simulink model "MIL_ASW"  (R2019b)
settings: Solver=FixedStepDiscrete  StartTime=0.0  StopTime=2  FixedStep=0.001  RelTol=1e-3  EnableMultiTasking=on
model workspace (MAT data in the model file):
  AccPedlCanVal : Simulink.Signal (value not decoded)
  AccPedlVal : Simulink.Signal (value not decoded)
  BrkPedlCanVal : Simulink.Signal (value not decoded)
  BrkPedlVal : Simulink.Signal (value not decoded)
  Cal1 : Simulink.Parameter (value not decoded)
  Cal10 : Simulink.Parameter (value not decoded)
  Cal11 : Simulink.Parameter (value not decoded)
  Cal12 : Simulink.Parameter (value not decoded)
  Cal2 : Simulink.Parameter (value not decoded)
  Cal3 : Simulink.Parameter (value not decoded)
  Cal4 : Simulink.Parameter (value not decoded)
  Cal5 : Simulink.Parameter (value not decoded)
  Cal6 : Simulink.Parameter (value not decoded)
  Cal7 : Simulink.Parameter (value not decoded)
  Cal8 : Simulink.Parameter (value not decoded)
  Cal9 : Simulink.Parameter (value not decoded)
  Clu1Act : Simulink.Signal (value not decoded)
  Clu1PTar : Simulink.Signal (value not decoded)
  Clu1Req : Simulink.Signal (value not decoded)
  Clu1TqTar : Simulink.Signal (value not decoded)
  Clu2Act : Simulink.Signal (value not decoded)
  Clu2PTar : Simulink.Signal (value not decoded)
  Clu2Req : Simulink.Signal (value not decoded)
  Clu2TqTar : Simulink.Signal (value not decoded)
  CluKissPtPLnch : Simulink.Parameter (value not decoded)
  CluOilTRawVal : Simulink.Signal (value not decoded)
  CluOilTVal : Simulink.Signal (value not decoded)
  CluOpenTqRatMax : Simulink.Parameter (value not decoded)
  CluPMap : Simulink.Parameter (value not decoded)
  CluPMax : Simulink.Parameter (value not decoded)
  CluPMaxGear1 : Simulink.Parameter (value not decoded)
  CluPMaxGear2 : Simulink.Parameter (value not decoded)
  CluPMaxGear3 : Simulink.Parameter (value not decoded)
  CluPMaxGear4 : Simulink.Parameter (value not decoded)
  CluPMaxGear5 : Simulink.Parameter (value not decoded)
  CluPMaxGear6 : Simulink.Parameter (value not decoded)
  CluPMaxGearR : Simulink.Parameter (value not decoded)
  CluPMin : Simulink.Parameter (value not decoded)
  CluPosnMax : Simulink.Parameter (value not decoded)
  CluSoln1IRawVal : Simulink.Signal (value not decoded)
  CluSoln1IReq : Simulink.Signal (value not decoded)
  CluSoln1IReqFlg : Simulink.Signal (value not decoded)
  CluSoln1IVal : Simulink.Signal (value not decoded)
  CluSoln1LineI : Simulink.Parameter (value not decoded)
  CluSoln1LineP : Simulink.Parameter (value not decoded)
  CluSoln1Pwm : Simulink.Signal (value not decoded)
  CluSoln2IRawVal : Simulink.Signal (value not decoded)
  CluSoln2IReq : Simulink.Signal (value not decoded)
  CluSoln2IReqFlg : Simulink.Signal (value not decoded)
  CluSoln2IVal : Simulink.Signal (value not decoded)
  CluSoln2LineI : Simulink.Parameter (value not decoded)
  CluSoln2LineP : Simulink.Parameter (value not decoded)
  CluSoln2Pwm : Simulink.Signal (value not decoded)
  CluTqMap : Simulink.Parameter (value not decoded)
  CrnkSpdRawVal : Simulink.Signal (value not decoded)
  CrnkSpdVal : Simulink.Signal (value not decoded)
  Drive_Intensity_Fuzzy : object (value not decoded)
  DrvIntenFzzy : Simulink.LookupTable (value not decoded)
  EngNIdle : Simulink.Parameter (value not decoded)
  EngNIdleMin : Simulink.Parameter (value not decoded)
  EngSpdCanVal : Simulink.Signal (value not decoded)
  EngThrCanVal : Simulink.Signal (value not decoded)
  EngTqAdd : Simulink.Parameter (value not decoded)
  EngTqCanVal : Simulink.Signal (value not decoded)
  EngTqIntvFlg : Simulink.Signal (value not decoded)
  EngTqIntvRat : Simulink.Signal (value not decoded)
  EngTqMapExtChartc : Simulink.Parameter (value not decoded)
  EngTqMapSpdIndx : Simulink.Parameter (value not decoded)
  EngTqMapThrtIndx : Simulink.Parameter (value not decoded)
  EngTqMapTqMax : Simulink.Parameter (value not decoded)
  EngTqMaxNorm : Simulink.Parameter (value not decoded)
  EngTqRef : Simulink.Parameter (value not decoded)
  EvenCluPRawVal : Simulink.Signal (value not decoded)
  EvenCluPVal : Simulink.Signal (value not decoded)
  EvenInpSpdRawVal : Simulink.Signal (value not decoded)
  EvenInpSpdVal : Simulink.Signal (value not decoded)
  FcnCallTime : Simulink.Parameter (value not decoded)
  FinalRat : Simulink.Parameter (value not decoded)
  Fork1A : Simulink.Parameter (value not decoded)
  Fork1Act : Simulink.Signal (value not decoded)
  Fork1B : Simulink.Parameter (value not decoded)
  Fork1DeltaSpdTar : Simulink.Parameter (value not decoded)
  Fork1MaxSpd1A : Simulink.Parameter (value not decoded)
  Fork1MaxSpd1B : Simulink.Parameter (value not decoded)
  Fork1MaxSpd2A : Simulink.Parameter (value not decoded)
  Fork1MaxSpd2B : Simulink.Parameter (value not decoded)
  Fork1PosnA : Simulink.Parameter (value not decoded)
  Fork1PosnB : Simulink.Parameter (value not decoded)
  Fork1PosnMaxSpd1A : Simulink.Parameter (value not decoded)
  Fork1PosnMaxSpd1B : Simulink.Parameter (value not decoded)
  Fork1PosnMaxSpd2A : Simulink.Parameter (value not decoded)
  Fork1PosnMaxSpd2B : Simulink.Parameter (value not decoded)
  Fork1PosnNeut : Simulink.Parameter (value not decoded)
  Fork1PosnNeutA : Simulink.Parameter (value not decoded)
  Fork1PosnNeutB : Simulink.Parameter (value not decoded)
  Fork1PosnRawVal : Simulink.Signal (value not decoded)
  Fork1PosnSyncA : Simulink.Parameter (value not decoded)
  Fork1PosnSyncB : Simulink.Parameter (value not decoded)
  Fork1PosnVal : Simulink.Signal (value not decoded)
  Fork1SyncTar : Simulink.Parameter (value not decoded)
  Fork2A : Simulink.Parameter (value not decoded)
  Fork2Act : Simulink.Signal (value not decoded)
  Fork2B : Simulink.Parameter (value not decoded)
  Fork2DeltaSpdTar : Simulink.Parameter (value not decoded)
  Fork2MaxSpd1A : Simulink.Parameter (value not decoded)
  Fork2MaxSpd1B : Simulink.Parameter (value not decoded)
  Fork2MaxSpd2A : Simulink.Parameter (value not decoded)
  Fork2MaxSpd2B : Simulink.Parameter (value not decoded)
  Fork2PosnA : Simulink.Parameter (value not decoded)
  Fork2PosnB : Simulink.Parameter (value not decoded)
  Fork2PosnMaxSpd1A : Simulink.Parameter (value not decoded)
  Fork2PosnMaxSpd1B : Simulink.Parameter (value not decoded)
  Fork2PosnMaxSpd2A : Simulink.Parameter (value not decoded)
  Fork2PosnMaxSpd2B : Simulink.Parameter (value not decoded)
  Fork2PosnNeut : Simulink.Parameter (value not decoded)
  Fork2PosnNeutA : Simulink.Parameter (value not decoded)
  Fork2PosnNeutB : Simulink.Parameter (value not decoded)
  Fork2PosnRawVal : Simulink.Signal (value not decoded)
  Fork2PosnSyncA : Simulink.Parameter (value not decoded)
  Fork2PosnSyncB : Simulink.Parameter (value not decoded)
  Fork2PosnVal : Simulink.Signal (value not decoded)
  Fork2SyncTar : Simulink.Parameter (value not decoded)
  Fork3A : Simulink.Parameter (value not decoded)
  Fork3Act : Simulink.Signal (value not decoded)
  Fork3B : Simulink.Parameter (value not decoded)
  Fork3DeltaSpdTar : Simulink.Parameter (value not decoded)
  Fork3MaxSpd1A : Simulink.Parameter (value not decoded)
  Fork3MaxSpd1B : Simulink.Parameter (value not decoded)
  Fork3MaxSpd2A : Simulink.Parameter (value not decoded)
  Fork3MaxSpd2B : Simulink.Parameter (value not decoded)
  Fork3PosnA : Simulink.Parameter (value not decoded)
  Fork3PosnB : Simulink.Parameter (value not decoded)
  Fork3PosnMaxSpd1A : Simulink.Parameter (value not decoded)
  Fork3PosnMaxSpd1B : Simulink.Parameter (value not decoded)
  Fork3PosnMaxSpd2A : Simulink.Parameter (value not decoded)
  Fork3PosnMaxSpd2B : Simulink.Parameter (value not decoded)
  Fork3PosnNeut : Simulink.Parameter (value not decoded)
  Fork3PosnNeutA : Simulink.Parameter (value not decoded)
  Fork3PosnNeutB : Simulink.Parameter (value not decoded)
  Fork3PosnRawVal : Simulink.Signal (value not decoded)
  Fork3PosnSyncA : Simulink.Parameter (value not decoded)
  Fork3PosnSyncB : Simulink.Parameter (value not decoded)
  Fork3PosnVal : Simulink.Signal (value not decoded)
  Fork3SyncTar : Simulink.Parameter (value not decoded)
  Fork4A : Simulink.Parameter (value not decoded)
  Fork4Act : Simulink.Signal (value not decoded)
  Fork4B : Simulink.Parameter (value not decoded)
  Fork4DeltaSpdTar : Simulink.Parameter (value not decoded)
  Fork4MaxSpd1A : Simulink.Parameter (value not decoded)
  Fork4MaxSpd1B : Simulink.Parameter (value not decoded)
  Fork4MaxSpd2A : Simulink.Parameter (value not decoded)
  Fork4MaxSpd2B : Simulink.Parameter (value not decoded)
  Fork4PosnA : Simulink.Parameter (value not decoded)
  Fork4PosnB : Simulink.Parameter (value not decoded)
  Fork4PosnMaxSpd1A : Simulink.Parameter (value not decoded)
  Fork4PosnMaxSpd1B : Simulink.Parameter (value not decoded)
  Fork4PosnMaxSpd2A : Simulink.Parameter (value not decoded)
  Fork4PosnMaxSpd2B : Simulink.Parameter (value not decoded)
  Fork4PosnNeut : Simulink.Parameter (value not decoded)
  Fork4PosnNeutA : Simulink.Parameter (value not decoded)
  Fork4PosnNeutB : Simulink.Parameter (value not decoded)
  Fork4PosnRawVal : Simulink.Signal (value not decoded)
  Fork4PosnSyncA : Simulink.Parameter (value not decoded)
  Fork4PosnSyncB : Simulink.Parameter (value not decoded)
  Fork4PosnVal : Simulink.Signal (value not decoded)
  Fork4SyncTar : Simulink.Parameter (value not decoded)
  FrntWhlRd : Simulink.Parameter (value not decoded)
  GearIdx : Simulink.Parameter (value not decoded)
  GearMax : Simulink.Parameter (value not decoded)
  GearRat : Simulink.Parameter (value not decoded)
  Launch_Engage_Fuzzy : object (value not decoded)
  LnchEngmtFzzy : Simulink.LookupTable (value not decoded)
  LubeSolnIRawVal : Simulink.Signal (value not decoded)
  LubeSolnIReq : Simulink.Signal (value not decoded)
  LubeSolnIVal : Simulink.Signal (value not decoded)
  LubeSolnLineI : Simulink.Parameter (value not decoded)
  LubeSolnLineP : Simulink.Parameter (value not decoded)
  LubeSolnPwm : Simulink.Signal (value not decoded)
  MaiLineSolnIRawVal : Simulink.Signal (value not decoded)
  MaiLineSolnIReq : Simulink.Signal (value not decoded)
  MaiLineSolnIVal : Simulink.Signal (value not decoded)
  MaiLineSolnLineI : Simulink.Parameter (value not decoded)
  MaiLineSolnLineP : Simulink.Parameter (value not decoded)
  MaiLineSolnPwm : Simulink.Signal (value not decoded)
  OddCluPRawVal : Simulink.Signal (value not decoded)
  OddCluPVal : Simulink.Signal (value not decoded)
  OddInpSpdRawVal : Simulink.Signal (value not decoded)
  OddInpSpdVal : Simulink.Signal (value not decoded)
  OutpSpdRawVal : Simulink.Signal (value not decoded)
  OutpSpdVal : Simulink.Signal (value not decoded)
  PsnsrLineP : Simulink.Parameter (value not decoded)
  PsnsrLineV : Simulink.Parameter (value not decoded)
  SftLvrCanVal : Simulink.Signal (value not decoded)
  SftLvrCfm : Simulink.Signal (value not decoded)
  SftLvrVal : Simulink.Signal (value not decoded)
  Shaft1GearAct : Simulink.Signal (value not decoded)
  Shaft1GearReq : Simulink.Signal (value not decoded)
  Shaft2GearAct : Simulink.Signal (value not decoded)
  Shaft2GearReq : Simulink.Signal (value not decoded)
  ShiftMux1SwtReq : Simulink.Signal (value not decoded)
  ShiftMux2SwtReq : Simulink.Signal (value not decoded)
  ShiftSdlEcoDwnSeln : Simulink.Parameter (value not decoded)
  ShiftSdlEcoDwnShift : Simulink.Parameter (value not decoded)
  ShiftSdlEcoUpSeln : Simulink.Parameter (value not decoded)
  ShiftSdlEcoUpShift : Simulink.Parameter (value not decoded)
  ShiftSdlPwrDwnSeln : Simulink.Parameter (value not decoded)
  ShiftSdlPwrDwnShift : Simulink.Parameter (value not decoded)
  ShiftSdlPwrUpSeln : Simulink.Parameter (value not decoded)
  ShiftSdlPwrUpShift : Simulink.Parameter (value not decoded)
  ShiftSdlSACDwnSeln : Simulink.Parameter (value not decoded)
  ShiftSdlSACDwnShift : Simulink.Parameter (value not decoded)
  ShiftSdlSACUpSeln : Simulink.Parameter (value not decoded)
  ShiftSdlSACUpShift : Simulink.Parameter (value not decoded)
  ShiftSdlThrPedlIdx : Simulink.Parameter (value not decoded)
  ShiftSoln1IRawVal : Simulink.Signal (value not decoded)
  ShiftSoln1IReq : Simulink.Signal (value not decoded)
  ShiftSoln1IVal : Simulink.Signal (value not decoded)
  ShiftSoln1LineI : Simulink.Parameter (value not decoded)
  ShiftSoln1LineP : Simulink.Parameter (value not decoded)
  ShiftSoln1Pwm : Simulink.Signal (value not decoded)
  ShiftSoln2IRawVal : Simulink.Signal (value not decoded)
  ShiftSoln2IReq : Simulink.Signal (value not decoded)
  ShiftSoln2IVal : Simulink.Signal (value not decoded)
  ShiftSoln2LineI : Simulink.Parameter (value not decoded)
  ShiftSoln2LineP : Simulink.Parameter (value not decoded)
  ShiftSoln2Pwm : Simulink.Signal (value not decoded)
  SolnOutpTRawVal : Simulink.Signal (value not decoded)
  SolnOutpTVal : Simulink.Signal (value not decoded)
  TSnsr1LineR : Simulink.Parameter (value not decoded)
  TSnsr2LineR : Simulink.Parameter (value not decoded)
  TrsmNrGearAct : Simulink.Signal (value not decoded)
  TrsmNrGearReq : Simulink.Signal (value not decoded)
  TrsmNrPreGearAct : Simulink.Signal (value not decoded)
  TrsmNrPreGearReq : Simulink.Signal (value not decoded)
  Tsnsr1LineT : Simulink.Parameter (value not decoded)
  Tsnsr2LineT : Simulink.Parameter (value not decoded)
  VehSpdCanVal : Simulink.Signal (value not decoded)
  VehSpdTrsmEstimd : Simulink.Signal (value not decoded)
  VehSpdVal : Simulink.Signal (value not decoded)
  VlvBodyTRawVal : Simulink.Signal (value not decoded)
  VlvBodyTVal : Simulink.Signal (value not decoded)
symbols that are objects in the model workspace (value not decoded): CluPMap, CluSoln1LineI, CluSoln1LineP, CluSoln2LineI, CluSoln2LineP, CluTqMap, EngNIdle, EngNIdleMin, EngTqMapThrtIndx, EngTqMapTqMax, EngTqMaxNorm, FcnCallTime, FinalRat, Fork1A, Fork1B, Fork1DeltaSpdTar, Fork1PosnA, Fork1PosnB, Fork1PosnMaxSpd1A, Fork1PosnMaxSpd1B, Fork1PosnMaxSpd2A, Fork1PosnMaxSpd2B, Fork1PosnNeut, Fork1PosnNeutA, Fork1PosnNeutB, Fork1PosnSyncA, Fork1PosnSyncB, Fork1SyncTar, Fork2A, Fork2B, Fork2DeltaSpdTar, Fork2PosnA, Fork2PosnB, Fork2PosnMaxSpd1A, Fork2PosnMaxSpd1B, Fork2PosnMaxSpd2A, Fork2PosnMaxSpd2B, Fork2PosnNeut, Fork2PosnNeutA, Fork2PosnNeutB, Fork2PosnSyncA, Fork2PosnSyncB, Fork2SyncTar, Fork3A, Fork3B, Fork3DeltaSpdTar, Fork3PosnA, Fork3PosnB, Fork3PosnMaxSpd1A, Fork3PosnMaxSpd1B, Fork3PosnMaxSpd2A, Fork3PosnMaxSpd2B, Fork3PosnNeut, Fork3PosnNeutA, Fork3PosnNeutB, Fork3PosnSyncA, Fork3PosnSyncB, Fork3SyncTar, Fork4A, Fork4B
undefined symbols (not defined in the file or in its folder): in1, out1
libraries: simulink x44, fuzblock x3
(part 7 of 10)

== stateflow chart MIL_ASW/Application_Software_SHAW/ASW_ClutchControl_new/Clutch_Control_Strategy ==
  state Inten=Driver_Intention_Fuzzy(AccPeld) [function] [commented out]
  state TqNew=Launch_Applied_Fuzzy(TqOld,Inten,EngN,CluN) [function]
  state Tq = Launch_Torque_Target(EngThr) [function]
  state Tq = Close_Torque_Target(EngThr) [function]
  state Odd_up_to_Even
    state Input [parallel]
      % states initialized
      en:
      Clu1Act=1;
      Clu2Act=0;
      Clu1PReqFlg=1;
      Clu2PReqFlg=1;
      Clu1TqTar=Clu1TqCpEstimd;
      Clu2TqTar=0;
      CluTqTarMin=0;
      CluTqTarMax=40000;
      % torque target initialized
      en:
      CluOffTqTar=Clu1TqTar;
      CluOnTqTar=Clu2TqTar;
      % speed allocation
      en,du:
      CluOffN=InpShaft1N;
      CluOnN=InpShaft2N;
      settings: executionOrder=1
      note: Shift from odd gear to even gear,
          | clutch 1 as off-going clutch,
          | clutch 2 as on-coming clutch
    state Main [parallel]
      settings: executionOrder=2
      state Phase_A
        %Preparation
        state Phase_A_On_Coming [parallel]
          settings: executionOrder=2
          state Phase_A_On_Coming1
            %Wait_for_KissPoint
            en:
            CluOnTqTar=1;
          (default) -> Odd_up_to_Even.Main.Phase_A.Phase_A_On_Coming.Phase_A_On_Coming1
        state Phase_A_Off_Going [parallel]
          settings: executionOrder=1
          state Phase_A_Off_Going1
            %release to slip
            en,du:
            CluTqTarMin=0;
            CluTqDec=1000;
            CluOffTqTar=max(CluOffTqTar-CluTqDec,CluTqTarMin);
          state Phase_A_Off_Going2
            en,du:
            CluTqTarMin=0;
            CluTqDec=100;
            CluOffTqTar=max(CluOffTqTar-CluTqDec,CluTqTarMin);
          state Phase_A_Off_Going3
          (default) -> Odd_up_to_Even.Main.Phase_A.Phase_A_Off_Going.Phase_A_Off_Going1
          Odd_up_to_Even.Main.Phase_A.Phase_A_Off_Going.Phase_A_Off_Going1 -> Odd_up_to_Even.Main.Phase_A.Phase_A_Off_Going.Phase_A_Off_Going2 : [CluOffTqTar<EngTq]
          Odd_up_to_Even.Main.Phase_A.Phase_A_Off_Going.Phase_A_Off_Going2 -> Odd_up_to_Even.Main.Phase_A.Phase_A_Off_Going.Phase_A_Off_Going3 : [abs(EngN-CluOffN)>10]
      state Phase_B_Power_on
        %Torque Phase, Handover
        state Phase_B_On_Coming [parallel]
          settings: executionOrder=1
          state Phase_B_On_Coming1
            en,du:
            CluTqTarMax=EngTq;
            CluTqInc=500;
            CluOnTqTar=min(CluOnTqTar+CluTqInc,CluTqTarMax);
          (default) -> Odd_up_to_Even.Main.Phase_B_Power_on.Phase_B_On_Coming.Phase_B_On_Coming1
        state Phase_B_Off_Going [parallel]
          settings: executionOrder=2
          state Phase_B_Off_Going1
            en,du:
            CluTqTarMin=0;
            CluTqDec=550;
            CluOffTqTar=max(CluOffTqTar-CluTqDec,CluTqTarMin);
          (default) -> Odd_up_to_Even.Main.Phase_B_Power_on.Phase_B_Off_Going.Phase_B_Off_Going1
      state Phase_B_Power_Off
        %Inertia Phase, Handover
        state Phase_B_Off_Going [parallel]
          settings: executionOrder=2
          state Phase_B_Off_Going1
            en,du:
            CluTqTarMin=0;
            CluTqDec=500;
            CluOffTqTar=max(CluOffTqTar-CluTqDec,CluTqTarMin);
          (default) -> Odd_up_to_Even.Main.Phase_B_Power_Off.Phase_B_Off_Going.Phase_B_Off_Going1
        state Phase_B_On_Coming [parallel]
          settings: executionOrder=1
          state Phase_B_On_Coming1
          (default) -> Odd_up_to_Even.Main.Phase_B_Power_Off.Phase_B_On_Coming.Phase_B_On_Coming1
      state Phase_C_Power_on
        %Inertia Phase
        en,du:
        CluTqTarMax=Close_Torque_Target(EngThr);
        CluTqInc=500;
        CluOnTqTar=min(CluOnTqTar+CluTqInc,CluTqTarMax);
      state Phase_C_Power_Off
        %Torque Phase
        en,du:
        CluTqTarMax=Close_Torque_Target(EngThr);
        CluTqInc=500;
        CluOnTqTar=min(CluOnTqTar+CluTqInc,CluTqTarMax);
      state Phase_D_Power_on
        %Synchronization Moment
        en,du:
        CluTqTarMax=Close_Torque_Target(EngThr);
        CluTqInc=500;
        CluOnTqTar=min(CluOnTqTar+CluTqInc,CluTqTarMax);
      state Phase_D_Power_Off
        %Synchronization Moment
        en,du:
        CluTqTarMax=Close_Torque_Target(EngThr);
        CluTqInc=500;
        CluOnTqTar=min(CluOnTqTar+CluTqInc,CluTqTarMax);
      state Phase_E_Power_on
        %Increae pressure for safety
        en,du:
        CluOnTqTar=min(CluOnTqTar+CluTqInc,CluTqTarMax);
        CluTqInc=1000;
        CluTqTarMax=Close_Torque_Target(EngThr);
      state Phase_E_Power_Off
        %Increae pressure for safety
        en,du:
        CluTqTarMax=Close_Torque_Target(EngThr);
        CluTqInc=1000;
        CluOnTqTar=min(CluOnTqTar+CluTqInc,CluTqTarMax);
      state End
      state End1
      (default) -> Odd_up_to_Even.Main.Phase_A
      Odd_up_to_Even.Main.Phase_A -> (junction 335) : [abs(EngN-CluOffN)>10]
      (junction 335) -> (junction 534) [order 2]
      (junction 335) -> Odd_up_to_Even.Main.Phase_B_Power_on [order 1] : [EngN>CluOffN]
          | %Power On
      (junction 534) -> Odd_up_to_Even.Main.Phase_B_Power_Off : %Power off
      Odd_up_to_Even.Main.Phase_B_Power_on -> Odd_up_to_Even.Main.Phase_C_Power_on : [CluOffTqTar<=0&&CluOnTqTar>=CluTqTarMax]
      Odd_up_to_Even.Main.Phase_B_Power_Off -> Odd_up_to_Even.Main.Phase_C_Power_Off : [CluOffTqTar<=0&&EngN<=CluOnN]
      Odd_up_to_Even.Main.Phase_C_Power_on -> Odd_up_to_Even.Main.Phase_D_Power_on : [abs(EngN-CluOnN)<50||...
          | EngN<=CluOnN]
      Odd_up_to_Even.Main.Phase_C_Power_Off -> Odd_up_to_Even.Main.Phase_D_Power_Off : [abs(EngN-CluOnN)<50]
      Odd_up_to_Even.Main.Phase_D_Power_on -> Odd_up_to_Even.Main.Phase_E_Power_on : [abs(EngN-CluOnN)<10]
      Odd_up_to_Even.Main.Phase_D_Power_Off -> Odd_up_to_Even.Main.Phase_E_Power_Off : [abs(EngN-CluOnN)<10]
      Odd_up_to_Even.Main.Phase_E_Power_Off -> Odd_up_to_Even.Main.End1 : [CluOnTqTar>=CluTqTarMax]
      Odd_up_to_Even.Main.Phase_E_Power_on -> Odd_up_to_Even.Main.End : [CluOnTqTar>=CluTqTarMax]
      Odd_up_to_Even.Main.End -> (junction 545)
      Odd_up_to_Even.Main.End1 -> (junction 546)
      (junction 545) -> (junction 546)
    state Output [parallel]
      en,du:
      Clu1TqTar=CluOffTqTar;
      Clu2TqTar=CluOnTqTar;
      settings: executionOrder=3
    (junction 546) -> (junction 859)
  state Odd_down_to_Even
    state Input [parallel]
      % states initialized
      en:
      Clu1Act=1;
      Clu2Act=0;
      Clu1PReqFlg=1;
      Clu2PReqFlg=1;
      Clu1TqTar=Clu1TqCpEstimd;
      Clu2TqTar=0;
      CluTqTarMin=0;
      CluTqTarMax=40000;
      % torque target initialized
      en:
      CluOffTqTar=Clu1TqTar;
      CluOnTqTar=Clu2TqTar;
      % speed allocation
      en,du:
      CluOffN=InpShaft1N;
      CluOnN=InpShaft2N;
      settings: executionOrder=1
      note: Shift from odd gear to even gear,
          | clutch 1 as off-going clutch,
          | clutch 2 as on-coming clutch
    state Main [parallel]
      settings: executionOrder=2
      state Phase_A
        %Preparation
        state Phase_A_Off_Going [parallel]
          settings: executionOrder=1
          state Phase_A_Off_Going1
            %release to slip
            en,du:
            CluTqTarMin=0;
            CluTqDec=1000;
            CluOffTqTar=max(CluOffTqTar-CluTqDec,CluTqTarMin);
          state Phase_A_Off_Going2
            en,du:
            CluTqTarMin=0;
            CluTqDec=100;
            CluOffTqTar=max(CluOffTqTar-CluTqDec,CluTqTarMin);
          state Phase_A_Off_Going3
          (default) -> Odd_down_to_Even.Main.Phase_A.Phase_A_Off_Going.Phase_A_Off_Going1
          Odd_down_to_Even.Main.Phase_A.Phase_A_Off_Going.Phase_A_Off_Going1 -> Odd_down_to_Even.Main.Phase_A.Phase_A_Off_Going.Phase_A_Off_Going2 : [CluOffTqTar<EngTq]
          Odd_down_to_Even.Main.Phase_A.Phase_A_Off_Going.Phase_A_Off_Going2 -> Odd_down_to_Even.Main.Phase_A.Phase_A_Off_Going.Phase_A_Off_Going3 : [abs(EngN-CluOffN)>10]
        state Phase_A_On_Coming [parallel]
          settings: executionOrder=2
          state Phase_A_On_Coming1
            %Wait_for_KissPoint
            en:
            CluOnTqTar=1;
          (default) -> Odd_down_to_Even.Main.Phase_A.Phase_A_On_Coming.Phase_A_On_Coming1
      state Phase_B_Power_on
        %Inertia Phase, Handover
        state Phase_B_Off_Going [parallel]
          settings: executionOrder=2
          state Phase_B_Off_Going1
            en,du:
            CluTqTarMin=0;
            CluTqDec=500;
            CluOffTqTar=max(CluOffTqTar-CluTqDec,CluTqTarMin);
          (default) -> Odd_down_to_Even.Main.Phase_B_Power_on.Phase_B_Off_Going.Phase_B_Off_Going1
        state Phase_B_On_Coming [parallel]
          settings: executionOrder=1
      state Phase_B_Power_Off
        %Torque Phase, Handover
        state Phase_B_Off_Going [parallel]
          settings: executionOrder=2
          state Phase_B_Off_Going1
            en,du:
            CluTqTarMin=0;
            CluTqDec=550;
            CluOffTqTar=max(CluOffTqTar-CluTqDec,CluTqTarMin);
          (default) -> Odd_down_to_Even.Main.Phase_B_Power_Off.Phase_B_Off_Going.Phase_B_Off_Going1
        state Phase_B_On_Coming [parallel]
          settings: executionOrder=1
          state Phase_B_On_Coming1
            en,du:
            CluTqTarMax=Close_Torque_Target(EngThr);
            CluTqInc=500;
            CluOnTqTar=min(CluOnTqTar+CluTqInc,CluTqTarMax);
          (default) -> Odd_down_to_Even.Main.Phase_B_Power_Off.Phase_B_On_Coming.Phase_B_On_Coming1
      state Phase_C_Power_on
        %Torque Phase
        state Phase_C_Off_Going [parallel]
          settings: executionOrder=1
          state Phase_C_Off_Going1
          state Phase_C_Off_Going2
            en,du:
            CluTqTarMin=0;
            CluTqDec=550;
            CluOffTqTar=max(CluOffTqTar-CluTqDec,CluTqTarMin);
          (default) -> Odd_down_to_Even.Main.Phase_C_Power_on.Phase_C_Off_Going.Phase_C_Off_Going1
          Odd_down_to_Even.Main.Phase_C_Power_on.Phase_C_Off_Going.Phase_C_Off_Going1 -> Odd_down_to_Even.Main.Phase_C_Power_on.Phase_C_Off_Going.Phase_C_Off_Going2 : [CluOffTqTar+CluOnTqTar>=EngTq]
        state Phase_C_On_Coming [parallel]
          settings: executionOrder=2
          state Phase_C_On_Coming1
            en,du:
            CluTqTarMax=Close_Torque_Target(EngThr);
            CluTqInc=500;
            CluOnTqTar=min(CluOnTqTar+CluTqInc,CluTqTarMax);
          (default) -> Odd_down_to_Even.Main.Phase_C_Power_on.Phase_C_On_Coming.Phase_C_On_Coming1
      state Phase_C_Power_Off
        %Inertia Phase
        en,du:
        CluTqTarMax=Close_Torque_Target(EngThr);
        CluTqInc=500;
        CluOnTqTar=min(CluOnTqTar+CluTqInc,CluTqTarMax);
      state Phase_D_Power_on
        %Synchronization Moment
        en,du:
        CluTqTarMax=Close_Torque_Target(EngThr);
        CluTqInc=500;
        CluOnTqTar=min(CluOnTqTar+CluTqInc,CluTqTarMax);
      state Phase_D_Power_Off
        %Synchronization Moment
        en,du:
        CluTqTarMax=Close_Torque_Target(EngThr);
        CluTqInc=500;
        CluOnTqTar=min(CluOnTqTar+CluTqInc,CluTqTarMax);
      state Phase_E_Power_on
        %Increae pressure for safety
        en,du:
        CluOnTqTar=min(CluOnTqTar+CluTqInc,CluTqTarMax);
        CluTqInc=1000;
        CluTqTarMax=Close_Torque_Target(EngThr);
      state Phase_E_Power_Off
        %Increae pressure for safety
        en,du:
        CluTqTarMax=Close_Torque_Target(EngThr);
        CluTqInc=1000;
        CluOnTqTar=min(CluOnTqTar+CluTqInc,CluTqTarMax);
      state End
      state End1
      (default) -> Odd_down_to_Even.Main.Phase_A
      Odd_down_to_Even.Main.Phase_A -> (junction 980) : [CluOffTqTar<=0||...
          | abs(EngN-CluOffN)>10]
      (junction 980) -> (junction 981) [order 2]
      (junction 980) -> Odd_down_to_Even.Main.Phase_B_Power_on [order 1] : [EngN>CluOffN]
          | %Power On
      (junction 981) -> Odd_down_to_Even.Main.Phase_B_Power_Off : %Power off
      Odd_down_to_Even.Main.Phase_B_Power_on -> Odd_down_to_Even.Main.Phase_B_Power_Off [order 2] : [EngTq<=0]
          | %change mind
          | % from power-on to power-off
      Odd_down_to_Even.Main.Phase_B_Power_on -> Odd_down_to_Even.Main.Phase_C_Power_on [order 1] : [EngN>CluOnN]
      Odd_down_to_Even.Main.Phase_B_Power_on -> Odd_down_to_Even.Main.Phase_C_Power_on [order 3] : after(100,tick)
      Odd_down_to_Even.Main.Phase_B_Power_Off -> Odd_down_to_Even.Main.Phase_C_Power_Off : [CluOffTqTar<=0]
      Odd_down_to_Even.Main.Phase_C_Power_Off -> Odd_down_to_Even.Main.Phase_D_Power_Off : [abs(EngN-CluOnN)<50]
      Odd_down_to_Even.Main.Phase_C_Power_on -> Odd_down_to_Even.Main.Phase_D_Power_on : [CluOffTqTar<=0&&...
          | abs(EngN-CluOnN)<50]
      Odd_down_to_Even.Main.Phase_D_Power_on -> Odd_down_to_Even.Main.Phase_E_Power_on : [abs(EngN-CluOnN)<10]
      Odd_down_to_Even.Main.Phase_D_Power_Off -> Odd_down_to_Even.Main.Phase_E_Power_Off : [abs(EngN-CluOnN)<10]
      Odd_down_to_Even.Main.Phase_E_Power_Off -> Odd_down_to_Even.Main.End1 : [CluOnTqTar>=CluTqTarMax]
      Odd_down_to_Even.Main.Phase_E_Power_on -> Odd_down_to_Even.Main.End : [CluOnTqTar>=CluTqTarMax]
      Odd_down_to_Even.Main.End -> (junction 982)
      Odd_down_to_Even.Main.End1 -> (junction 954)
      (junction 982) -> (junction 954)
    state Output [parallel]
      en,du:
      Clu1TqTar=CluOffTqTar;
      Clu2TqTar=CluOnTqTar;
      settings: executionOrder=3
    (junction 954) -> (junction 1009)
  state Both_Off_from_Odd2Even
    state Initial
      en:
      Clu1Act=1;
      Clu2Act=0;
      Clu1PReqFlg=1;
      Clu2PReqFlg=1;
      Clu1TqTar=Clu1TqCpEstimd;
      Clu2TqTar=Clu2TqCpEstimd;
    state Phase_A
      state Phase_A_Odd [parallel]
        settings: executionOrder=1
        state Phase_A_Odd
          %release to slip
          en,du:
          CluTqTarMin=0;
          CluTqDec=1000;
          Clu1TqTar=max(Clu1TqTar-CluTqDec,CluTqTarMin);
        state Phase_A_Odd1
          %release clutch
          en,du:
          CluTqTarMin=0;
          CluTqDec=500;
          Clu1TqTar=max(Clu1TqTar-CluTqDec,CluTqTarMin);
        state End
        (default) -> Both_Off_from_Odd2Even.Phase_A.Phase_A_Odd.Phase_A_Odd
        Both_Off_from_Odd2Even.Phase_A.Phase_A_Odd.Phase_A_Odd -> Both_Off_from_Odd2Even.Phase_A.Phase_A_Odd.Phase_A_Odd1 : [abs(EngN-InpShaft1N)>10]
        Both_Off_from_Odd2Even.Phase_A.Phase_A_Odd.Phase_A_Odd1 -> Both_Off_from_Odd2Even.Phase_A.Phase_A_Odd.End : [Clu1TqTar<=0]
      state Phase_A_Even [parallel]
        settings: executionOrder=2
        state Phase_A_Even
          %release to slip
          en,du:
          CluTqTarMin=0;
          CluTqDec=1000;
          Clu2TqTar=max(Clu2TqTar-CluTqDec,CluTqTarMin);
        state Phase_A_Even1
          %release clutch
          en,du:
          CluTqTarMin=0;
          CluTqDec=500;
          Clu2TqTar=max(Clu2TqTar-CluTqDec,CluTqTarMin);
        state End
        (default) -> Both_Off_from_Odd2Even.Phase_A.Phase_A_Even.Phase_A_Even
        Both_Off_from_Odd2Even.Phase_A.Phase_A_Even.Phase_A_Even -> Both_Off_from_Odd2Even.Phase_A.Phase_A_Even.Phase_A_Even1 : [abs(EngN-InpShaft2N)>10]
        Both_Off_from_Odd2Even.Phase_A.Phase_A_Even.Phase_A_Even1 -> Both_Off_from_Odd2Even.Phase_A.Phase_A_Even.End : [Clu2TqTar<=0]
    state End
    (default) -> Both_Off_from_Odd2Even.Initial
    Both_Off_from_Odd2Even.Initial -> Both_Off_from_Odd2Even.Phase_A
    Both_Off_from_Odd2Even.Phase_A -> Both_Off_from_Odd2Even.End : [Clu1TqTar<=0&&Clu2TqTar<=0]
  state Drive_by_Even
    state Initial
      en:
      Clu1Act=0;
      Clu2Act=1;
      Clu1PReqFlg=0;
      Clu2PReqFlg=1;
      Clu1TqTar=0;
      du:
      CluTqTarMax=Close_Torque_Target(EngThr);
      Clu2TqTar=max(Clu2TqTar,CluTqTarMax);
    (default) -> Drive_by_Even.Initial
  state Drive_by_Odd
    state Initial
      en:
      Clu1Act=1;
      Clu2Act=0;
      Clu1PReqFlg=1;
      Clu2PReqFlg=0;
      Clu2TqTar=0;
      du:
      CluTqTarMax=Close_Torque_Target(EngThr);
      Clu1TqTar=max(Clu1TqTar,CluTqTarMax);
    (default) -> Drive_by_Odd.Initial
  state Odd_Off
    state Initial
      en:
      Clu1Act=1;
      Clu2Act=0;
      Clu1PReqFlg=1;
      Clu2PReqFlg=0;
      Clu1TqTar=Clu1TqCpEstimd;
      Clu2TqTar=0;
    state Phase_A
      %release to slip
      en,du:
      CluTqTarMin=0;
      CluTqDec=1000;
      Clu1TqTar=max(Clu1TqTar-CluTqDec,CluTqTarMin);
    state Phase_B
      %release clutch
      en,du:
      CluTqTarMin=0;
      CluTqDec=500;
      Clu1TqTar=max(Clu1TqTar-CluTqDec,CluTqTarMin);
    state End
    (default) -> Odd_Off.Initial
    Odd_Off.Initial -> Odd_Off.Phase_A
    Odd_Off.Phase_A -> Odd_Off.Phase_B : [abs(EngN-InpShaft1N)>10]
    Odd_Off.Phase_B -> Odd_Off.End : [Clu1TqTar<=0]
  state Both_Clutch_Off
    state Keep_Both_off
      en:
      Clu1Act=0;
      Clu2Act=0;
      Clu1PReqFlg=0;
      Clu2PReqFlg=0;
      Clu1TqTar=0;
      Clu2TqTar=0;
      EngTqIntvFlg=0;
      EngTqIntvRat=100;
    (default) -> Keep_Both_off
  state Even_Off
    state Initial
      en:
      Clu1Act=0;
      Clu2Act=1;
      Clu1PReqFlg=0;
      Clu2PReqFlg=1;
      Clu1TqTar=0;
      Clu2TqTar=Clu2TqCpEstimd;
    state Phase_A
      %release to slip
      en,du:
      CluTqTarMin=0;
      CluTqDec=1000;
      Clu2TqTar=max(Clu2TqTar-CluTqDec,CluTqTarMin);
    state Phase_B
      %release clutch
      en,du:
      CluTqTarMin=0;
      CluTqDec=500;
      Clu2TqTar=max(Clu2TqTar-CluTqDec,CluTqTarMin);
    state End
    (default) -> Even_Off.Initial
    Even_Off.Initial -> Even_Off.Phase_A
    Even_Off.Phase_A -> Even_Off.Phase_B : [abs(EngN-InpShaft2N)>10]
    Even_Off.Phase_B -> Even_Off.End : [Clu2TqTar<=0]
  state Odd_On_Process
    state Odd_On
      state Initial
        en:
        Clu1Act=0;
        Clu2Act=0;
        Clu1PReqFlg=1;
        Clu2PReqFlg=0;
        Clu1TqTar=0;
        Clu2TqTar=0;
        CluTqTarMin=0;
        CluTqTarMax=40000;
      state Phase_A
        %Preparation
        %Wait_for_KissPoint
        en:
        Clu1TqTar=1;
      state Phase_B
        %Torque applied
        en,du:
        CluTqTarMax=Close_Torque_Target(EngThr);
        CluTqInc=500;
        Clu1TqTar=min(Clu1TqTar+CluTqInc,CluTqTarMax);
      state Phase_C
        %Synchronization
        en,du:
        CluTqTarMax=Close_Torque_Target(EngThr);
        CluTqInc=500;
        Clu1TqTar=Clu1TqTar+CluTqInc;
      state Phase_D
        %Increae pressure for safety
        en,du:
        CluTqTarMax=Close_Torque_Target(EngThr);
        CluTqInc=1000;
        Clu1TqTar=Clu1TqTar+CluTqInc;
      state End
      (default) -> Odd_On_Process.Odd_On.Initial
      Odd_On_Process.Odd_On.Initial -> Odd_On_Process.Odd_On.Phase_A
      Odd_On_Process.Odd_On.Phase_A -> Odd_On_Process.Odd_On.Phase_B : %[Clu1TqCpEstimd>0]
      Odd_On_Process.Odd_On.Phase_B -> Odd_On_Process.Odd_On.Phase_C : [abs(EngN-InpShaft1N)<50]
      Odd_On_Process.Odd_On.Phase_C -> Odd_On_Process.Odd_On.Phase_D : [abs(EngN-InpShaft1N)<10]
      Odd_On_Process.Odd_On.Phase_D -> Odd_On_Process.Odd_On.End : [Clu1TqTar>=CluTqTarMax]
    state Odd_Launch
      state Initial
        en:
        Clu1Act=0;
        Clu2Act=0;
        Clu1PReqFlg=1;
        Clu2PReqFlg=0;
        Clu1TqTar=0;
        Clu2TqTar=0;
        CluTqTarMin=0;
        CluTqTarMax=40000;
      state Phase_A
        %Preparation
        %Wait_for_KissPoint
        en:
        Clu1TqTar=1;
      state Phase_A1
        %Preparation
        %Wait_for_KissPoint
        en:
        Clu1TqTar=1;
      state Phase_B
        %Torque applied
        en,du:
        CluTqTarMax=Launch_Torque_Target(EngThr);
        %DrvrInten=Driver_Intention_Fuzzy(AccPedl);
        Clu1TqTar=Launch_Applied_Fuzzy(Clu1TqTar,DrvrInten,EngN,InpShaft1N);
        Clu1TqTar=min(Clu1TqTar,CluTqTarMax);
        %CluTqInc=20;
        %Clu1TqTar=min(Clu1TqTar+CluTqInc,CluTqTarMax);
      state Phase_B1
        %Torque applied
        en,du:
        CluTqTarMax=Launch_Torque_Target(EngThr);
        Clu1TqTar=Launch_Applied_Fuzzy(Clu1TqTar,DrvrInten,EngN,InpShaft1N);
        Clu1TqTar=min(Clu1TqTar,CluTqTarMax);
      state Phase_C1
        %Synchronization
        en,du:
        CluTqTarMax=Launch_Torque_Target(EngThr);
        CluTqInc=500;
        Clu1TqTar=Clu1TqTar+CluTqInc;
      state Phase_C
        %Synchronization
        en,du:
        CluTqTarMax=Launch_Torque_Target(EngThr);
        CluTqInc=500;
        Clu1TqTar=Clu1TqTar+CluTqInc;
      state Phase_D
        %Increae pressure for safety
        en,du:
        CluTqTarMax=Launch_Torque_Target(EngThr);
        CluTqInc=1000;
        Clu1TqTar=Clu1TqTar+CluTqInc;
      state Phase_D1
        %Increae pressure for safety
        en,du:
        CluTqTarMax=Launch_Torque_Target(EngThr);
        CluTqInc=1000;
        Clu1TqTar=Clu1TqTar+CluTqInc;
      state End
      state End1
      (default) -> Odd_On_Process.Odd_Launch.Initial
      Odd_On_Process.Odd_Launch.Initial -> Odd_On_Process.Odd_Launch.Phase_A [order 1] : %Static_Launch
          | [VehSpd<200]
      Odd_On_Process.Odd_Launch.Initial -> Odd_On_Process.Odd_Launch.Phase_A1 [order 2] : %Motion_Launch
      Odd_On_Process.Odd_Launch.Phase_A -> Odd_On_Process.Odd_Launch.Phase_B : %[InpShaft1N>0]
      Odd_On_Process.Odd_Launch.Phase_A1 -> Odd_On_Process.Odd_Launch.Phase_B1 : %[InpShaft1N>0]
      Odd_On_Process.Odd_Launch.Phase_B -> Odd_On_Process.Odd_Launch.Phase_C : [EngN>=EngNIdle &&...
          | abs(EngN-InpShaft1N)<50]
      Odd_On_Process.Odd_Launch.Phase_B1 -> Odd_On_Process.Odd_Launch.Phase_C1 : [EngN>=EngNIdle &&...
          | abs(EngN-InpShaft1N)<50]
      Odd_On_Process.Odd_Launch.Phase_C -> Odd_On_Process.Odd_Launch.Phase_D : [abs(EngN-InpShaft1N)<10]
      Odd_On_Process.Odd_Launch.Phase_C1 -> Odd_On_Process.Odd_Launch.Phase_D1 : [abs(EngN-InpShaft1N)<10]
      Odd_On_Process.Odd_Launch.Phase_D -> Odd_On_Process.Odd_Launch.End : [Clu1TqTar>=CluTqTarMax]
      Odd_On_Process.Odd_Launch.Phase_D1 -> Odd_On_Process.Odd_Launch.End1 : [Clu1TqTar>=CluTqTarMax]
      Odd_On_Process.Odd_Launch.End -> (junction 137)
      Odd_On_Process.Odd_Launch.End1 -> (junction 137)
    state Reverse_Launch
      state Initial
        en:
        Clu1Act=0;
        Clu2Act=0;
        Clu1PReqFlg=1;
        Clu2PReqFlg=0;
        Clu1TqTar=0;
        Clu2TqTar=0;
        CluTqTarMin=0;
        CluTqTarMax=40000;
      state Phase_A
        %Preparation
        %Wait_for_KissPoint
        en:
        Clu1TqTar=1;
      state Phase_A1
        %Preparation
        %Wait_for_KissPoint
        en:
        Clu1TqTar=1;
      state Phase_B
        %Torque applied
        en,du:
        CluTqTarMax=Launch_Torque_Target(EngThr);
        Clu1TqTar=Launch_Applied_Fuzzy(Clu1TqTar,DrvrInten,EngN,InpShaft1N);
        Clu1TqTar=min(Clu1TqTar,CluTqTarMax);
      state Phase_B1
        %Torque applied
        en,du:
        CluTqTarMax=Launch_Torque_Target(EngThr);
        Clu1TqTar=Launch_Applied_Fuzzy(Clu1TqTar,DrvrInten,EngN,InpShaft1N);
        Clu1TqTar=min(Clu1TqTar,CluTqTarMax);
      state Phase_C
        %Synchronization
        en,du:
        CluTqTarMax=Close_Torque_Target(EngThr);
        CluTqInc=500;
        Clu1TqTar=Clu1TqTar+CluTqInc;
      state Phase_C1
        %Synchronization
        en,du:
        CluTqTarMax=Close_Torque_Target(EngThr);
        CluTqInc=500;
        Clu1TqTar=Clu1TqTar+CluTqInc;
      state Phase_D
        %Increae pressure for safety
        en,du:
        CluTqTarMax=Launch_Torque_Target(EngThr);
        CluTqInc=1000;
        Clu1TqTar=Clu1TqTar+CluTqInc;
      state Phase_D1
        %Increae pressure for safety
        en,du:
        CluTqTarMax=Launch_Torque_Target(EngThr);
        CluTqInc=1000;
        Clu1TqTar=Clu1TqTar+CluTqInc;
      state End
      state End1
      (default) -> Odd_On_Process.Reverse_Launch.Initial
      Odd_On_Process.Reverse_Launch.Initial -> Odd_On_Process.Reverse_Launch.Phase_A [order 1] : %Static_Launch
          | [VehSpd<200]
      Odd_On_Process.Reverse_Launch.Initial -> Odd_On_Process.Reverse_Launch.Phase_A1 [order 2] : %Motion_Launch
      Odd_On_Process.Reverse_Launch.Phase_A -> Odd_On_Process.Reverse_Launch.Phase_B : %[InpShaft1N>0]
      Odd_On_Process.Reverse_Launch.Phase_A1 -> Odd_On_Process.Reverse_Launch.Phase_B1 : %[InpShaft1N>0]
      Odd_On_Process.Reverse_Launch.Phase_B -> Odd_On_Process.Reverse_Launch.Phase_C : [EngN>=EngNIdle &&...
          | abs(EngN-InpShaft1N)<50]
      Odd_On_Process.Reverse_Launch.Phase_B1 -> Odd_On_Process.Reverse_Launch.Phase_C1 : [EngN>=EngNIdle &&...
          | abs(EngN-InpShaft1N)<50]
      Odd_On_Process.Reverse_Launch.Phase_C1 -> Odd_On_Process.Reverse_Launch.Phase_D1 : [abs(EngN-InpShaft1N)<10]
      Odd_On_Process.Reverse_Launch.Phase_C -> Odd_On_Process.Reverse_Launch.Phase_D : [abs(EngN-InpShaft1N)<10]
      Odd_On_Process.Reverse_Launch.Phase_D -> Odd_On_Process.Reverse_Launch.End : [Clu1TqTar>=CluTqTarMax]
      Odd_On_Process.Reverse_Launch.Phase_D1 -> Odd_On_Process.Reverse_Launch.End1 : [Clu1TqTar>=CluTqTarMax]
      Odd_On_Process.Reverse_Launch.End -> (junction 273)
      Odd_On_Process.Reverse_Launch.End1 -> (junction 273)
  state Even_On_Process
    state Even_On
      state Initial
        en:
        Clu1Act=0;
        Clu2Act=0;
        Clu1PReqFlg=0;
        Clu2PReqFlg=1;
        Clu1TqTar=0;
        Clu2TqTar=0;
        CluTqTarMin=0;
        CluTqTarMax=40000;
      state Phase_A
        %Preparation
        %Wait_for_KissPoint
        en:
        Clu2TqTar=1;
      state Phase_B
        %Torque applied
        en,du:
        CluTqTarMax=Close_Torque_Target(EngThr);
        CluTqInc=500;
        Clu2TqTar=min(Clu2TqTar+CluTqInc,CluTqTarMax);
      state Phase_C
        %Synchronization
        en,du:
        CluTqTarMax=Close_Torque_Target(EngThr);
        CluTqInc=500;
        Clu2TqTar=Clu2TqTar+CluTqInc;
      state Phase_D
        %Increae pressure for safety
        en,du:
        CluTqTarMax=Close_Torque_Target(EngThr);
        CluTqInc=1000;
        Clu2TqTar=Clu2TqTar+CluTqInc;
      state End
      (default) -> Even_On_Process.Even_On.Initial
      Even_On_Process.Even_On.Initial -> Even_On_Process.Even_On.Phase_A
      Even_On_Process.Even_On.Phase_A -> Even_On_Process.Even_On.Phase_B : %[Clu2TqCpEstimd>0]
      Even_On_Process.Even_On.Phase_B -> Even_On_Process.Even_On.Phase_C : [abs(EngN-InpShaft2N)<50]
      Even_On_Process.Even_On.Phase_C -> Even_On_Process.Even_On.Phase_D : [abs(EngN-InpShaft2N)<10]
      Even_On_Process.Even_On.Phase_D -> Even_On_Process.Even_On.End : [Clu2TqTar>=CluTqTarMax]
    state Even_Launch
      state Initial
        en:
        Clu1Act=0;
        Clu2Act=0;
        Clu1PReqFlg=0;
        Clu2PReqFlg=1;
        Clu1TqTar=0;
        Clu2TqTar=0;
        CluTqTarMin=0;
        CluTqTarMax=40000;
      state Phase_A
        %Preparation
        %Wait_for_KissPoint
        en:
        Clu2TqTar=1;
      state Phase_A1
        %Preparation
        %Wait_for_KissPoint
        en:
        Clu2TqTar=1;
      state Phase_B
        %Torque applied
        en,du:
        CluTqTarMax=Launch_Torque_Target(EngThr);
        Clu2TqTar=Launch_Applied_Fuzzy(Clu2TqTar,DrvrInten,EngN,InpShaft2N);
        Clu2TqTar=min(Clu2TqTar,CluTqTarMax);
      state Phase_B1
        %Torque applied
        en,du:
        CluTqTarMax=Launch_Torque_Target(EngThr);
        Clu2TqTar=Launch_Applied_Fuzzy(Clu2TqTar,DrvrInten,EngN,InpShaft2N);
        Clu2TqTar=min(Clu2TqTar+CluTqInc,CluTqTarMax);
      state Phase_C1
        %Synchronization
        en,du:
        CluTqTarMax=Launch_Torque_Target(EngThr);
        CluTqInc=500;
        Clu2TqTar=Clu2TqTar+CluTqInc;
      state Phase_C
        %Synchronization
        en,du:
        CluTqTarMax=Launch_Torque_Target(EngThr);
        CluTqInc=500;
        Clu2TqTar=Clu2TqTar+CluTqInc;
      state Phase_D
        %Increae pressure for safety
        en,du:
        CluTqTarMax=Launch_Torque_Target(EngThr);
        CluTqInc=1000;
        Clu2TqTar=Clu2TqTar+CluTqInc;
      state Phase_D1
        %Increae pressure for safety
        en,du:
        CluTqTarMax=Launch_Torque_Target(EngThr);
        CluTqInc=1000;
        Clu2TqTar=Clu2TqTar+CluTqInc;
      state End
      state End1
      (default) -> Even_On_Process.Even_Launch.Initial
      Even_On_Process.Even_Launch.Initial -> Even_On_Process.Even_Launch.Phase_A [order 1] : %Static_Launch
          | [VehSpd<200]
      Even_On_Process.Even_Launch.Initial -> Even_On_Process.Even_Launch.Phase_A1 [order 2] : %Motion_Launch
      Even_On_Process.Even_Launch.Phase_A -> Even_On_Process.Even_Launch.Phase_B : %[InpShaft2N>0]
      Even_On_Process.Even_Launch.Phase_A1 -> Even_On_Process.Even_Launch.Phase_B1 : %[InpShaft2N>0]
      Even_On_Process.Even_Launch.Phase_B -> Even_On_Process.Even_Launch.Phase_C : [EngN>=EngNIdle &&...
          | abs(EngN-InpShaft2N)<50]
      Even_On_Process.Even_Launch.Phase_B1 -> Even_On_Process.Even_Launch.Phase_C1 : [EngN>=EngNIdle &&...
          | abs(EngN-InpShaft2N)<50]
      Even_On_Process.Even_Launch.Phase_C -> Even_On_Process.Even_Launch.Phase_D : [abs(EngN-InpShaft2N)<10]
      Even_On_Process.Even_Launch.Phase_C1 -> Even_On_Process.Even_Launch.Phase_D1 : [abs(EngN-InpShaft1N)<10]
      Even_On_Process.Even_Launch.Phase_D -> Even_On_Process.Even_Launch.End : [Clu2TqTar>=CluTqTarMax]
      Even_On_Process.Even_Launch.Phase_D1 -> Even_On_Process.Even_Launch.End1 : [Clu2TqTar>=CluTqTarMax]
      Even_On_Process.Even_Launch.End -> (junction 428)
      Even_On_Process.Even_Launch.End1 -> (junction 428)
  state Both_Off_from_Even2Odd
    state Initial
      en:
      Clu1Act=0;
      Clu2Act=1;
      Clu1PReqFlg=1;
      Clu2PReqFlg=1;
      Clu1TqTar=Clu1TqCpEstimd;
      Clu2TqTar=Clu2TqCpEstimd;
    state Phase_A
      state Phase_A_Odd [parallel]
        settings: executionOrder=1
        state Phase_A_Odd
          %release to slip
          en,du:
          CluTqTarMin=0;
          CluTqDec=1000;
          Clu1TqTar=max(Clu1TqTar-CluTqDec,CluTqTarMin);
        state Phase_A_Odd1
          %release clutch
          en,du:
          CluTqTarMin=0;
          CluTqDec=500;
          Clu1TqTar=max(Clu1TqTar-CluTqDec,CluTqTarMin);
        state End
        (default) -> Both_Off_from_Even2Odd.Phase_A.Phase_A_Odd.Phase_A_Odd
        Both_Off_from_Even2Odd.Phase_A.Phase_A_Odd.Phase_A_Odd -> Both_Off_from_Even2Odd.Phase_A.Phase_A_Odd.Phase_A_Odd1 : [abs(EngN-InpShaft1N)>10]
        Both_Off_from_Even2Odd.Phase_A.Phase_A_Odd.Phase_A_Odd1 -> Both_Off_from_Even2Odd.Phase_A.Phase_A_Odd.End : [Clu1TqTar<=0]
      state Phase_A_Even [parallel]
        settings: executionOrder=2
        state Phase_A_Even
          %release to slip
          en,du:
          CluTqTarMin=0;
          CluTqDec=1000;
          Clu2TqTar=max(Clu2TqTar-CluTqDec,CluTqTarMin);
        state Phase_A_Even1
          %release clutch
          en,du:
          CluTqTarMin=0;
          CluTqDec=500;
          Clu2TqTar=max(Clu2TqTar-CluTqDec,CluTqTarMin);
        state End
        (default) -> Both_Off_from_Even2Odd.Phase_A.Phase_A_Even.Phase_A_Even
        Both_Off_from_Even2Odd.Phase_A.Phase_A_Even.Phase_A_Even -> Both_Off_from_Even2Odd.Phase_A.Phase_A_Even.Phase_A_Even1 : [abs(EngN-InpShaft2N)>10]
        Both_Off_from_Even2Odd.Phase_A.Phase_A_Even.Phase_A_Even1 -> Both_Off_from_Even2Odd.Phase_A.Phase_A_Even.End : [Clu2TqTar<=0]
    state End
    (default) -> Both_Off_from_Even2Odd.Initial
    Both_Off_from_Even2Odd.Initial -> Both_Off_from_Even2Odd.Phase_A
    Both_Off_from_Even2Odd.Phase_A -> Both_Off_from_Even2Odd.End : [Clu1TqTar<=0&&Clu2TqTar<=0]
  state Even_up_to_Odd
    state Input [parallel]
      % states initialized
      en:
      Clu1Act=0;
      Clu2Act=1;
      Clu1PReqFlg=1;
      Clu2PReqFlg=1;
      Clu1TqTar=0;
      Clu2TqTar=Clu2TqCpEstimd;
      CluTqTarMin=0;
      CluTqTarMax=40000;
      % torque target initialized
      en:
      CluOffTqTar=Clu2TqTar;
      CluOnTqTar=Clu1TqTar;
      % speed allocation
      en,du:
      CluOffN=InpShaft2N;
      CluOnN=InpShaft1N;
      settings: executionOrder=1
      note: Shift from even gear to odd gear,
          | clutch 1 as on-coming clutch,
          | clutch 2 as off-going clutch
    state Main [parallel]
      settings: executionOrder=2
      state Phase_A
        %Preparation
        state Phase_A_Off_Going [parallel]
          settings: executionOrder=1
          state Phase_A_Off_Going1
            %release to slip
            en,du:
            CluTqTarMin=0;
            CluTqDec=1000;
            CluOffTqTar=max(CluOffTqTar-CluTqDec,CluTqTarMin);
          state Phase_A_Off_Going2
            en,du:
            CluTqTarMin=0;
            CluTqDec=100;
            CluOffTqTar=max(CluOffTqTar-CluTqDec,CluTqTarMin);
          state Phase_A_Off_Going3
          (default) -> Even_up_to_Odd.Main.Phase_A.Phase_A_Off_Going.Phase_A_Off_Going1
          Even_up_to_Odd.Main.Phase_A.Phase_A_Off_Going.Phase_A_Off_Going1 -> Even_up_to_Odd.Main.Phase_A.Phase_A_Off_Going.Phase_A_Off_Going2 : [CluOffTqTar<EngTq]
          Even_up_to_Odd.Main.Phase_A.Phase_A_Off_Going.Phase_A_Off_Going2 -> Even_up_to_Odd.Main.Phase_A.Phase_A_Off_Going.Phase_A_Off_Going3 : [abs(EngN-CluOffN)>10]
        state Phase_A_On_Coming [parallel]
          settings: executionOrder=2
          state Phase_A_On_Coming1
            %Wait_for_KissPoint
            en:
            CluOnTqTar=1;
          (default) -> Even_up_to_Odd.Main.Phase_A.Phase_A_On_Coming.Phase_A_On_Coming1
      state Phase_B_Power_on
        %Torque Phase, Handover
        state Phase_B_On_Coming [parallel]
          settings: executionOrder=1
          state Phase_B_On_Coming1
            en,du:
            CluTqTarMax=EngTq;
            CluTqInc=500;
            CluOnTqTar=min(CluOnTqTar+CluTqInc,CluTqTarMax);
          (default) -> Even_up_to_Odd.Main.Phase_B_Power_on.Phase_B_On_Coming.Phase_B_On_Coming1
        state Phase_B_Off_Going [parallel]
          settings: executionOrder=2
          state Phase_B_Off_Going1
            en,du:
            CluTqTarMin=0;
            CluTqDec=550;
            CluOffTqTar=max(CluOffTqTar-CluTqDec,CluTqTarMin);
          (default) -> Even_up_to_Odd.Main.Phase_B_Power_on.Phase_B_Off_Going.Phase_B_Off_Going1
      state Phase_B_Power_Off
        %Inertia Phase, Handover
        state Phase_B_Off_Going [parallel]
          settings: executionOrder=2
          state Phase_B_Off_Going1
            en,du:
            CluTqTarMin=0;
            CluTqDec=500;
            CluOffTqTar=max(CluOffTqTar-CluTqDec,CluTqTarMin);
          (default) -> Even_up_to_Odd.Main.Phase_B_Power_Off.Phase_B_Off_Going.Phase_B_Off_Going1
        state Phase_B_On_Coming [parallel]
          settings: executionOrder=1
          state Phase_B_On_Coming1
          (default) -> Even_up_to_Odd.Main.Phase_B_Power_Off.Phase_B_On_Coming.Phase_B_On_Coming1
      state Phase_C_Power_on
        %Inertia Phase
        en,du:
        CluTqTarMax=Close_Torque_Target(EngThr);
        CluTqInc=500;
        CluOnTqTar=min(CluOnTqTar+CluTqInc,CluTqTarMax);
      state Phase_C_Power_Off
        %Torque Phase
        en,du:
        CluTqTarMax=Close_Torque_Target(EngThr);
        CluTqInc=500;
        CluOnTqTar=min(CluOnTqTar+CluTqInc,CluTqTarMax);
      state Phase_D_Power_on
        %Synchronization Moment
        en,du:
        CluTqTarMax=Close_Torque_Target(EngThr);
        CluTqInc=500;
        CluOnTqTar=min(CluOnTqTar+CluTqInc,CluTqTarMax);
      state Phase_D_Power_Off
        %Synchronization Moment
        en,du:
        CluTqTarMax=Close_Torque_Target(EngThr);
        CluTqInc=500;
        CluOnTqTar=min(CluOnTqTar+CluTqInc,CluTqTarMax);
      state Phase_E_Power_on
        %Increae pressure for safety
        en,du:
        CluOnTqTar=min(CluOnTqTar+CluTqInc,CluTqTarMax);
        CluTqInc=1000;
        CluTqTarMax=Close_Torque_Target(EngThr);
      state Phase_E_Power_Off
        %Increae pressure for safety
        en,du:
        CluTqTarMax=Close_Torque_Target(EngThr);
        CluTqInc=1000;
        CluOnTqTar=min(CluOnTqTar+CluTqInc,CluTqTarMax);
      state End
      state End1
      (default) -> Even_up_to_Odd.Main.Phase_A
      Even_up_to_Odd.Main.Phase_A -> (junction 912) : [abs(EngN-CluOffN)>10]
      (junction 912) -> (junction 913) [order 2]
      (junction 912) -> Even_up_to_Odd.Main.Phase_B_Power_on [order 1] : [EngN>CluOffN]
          | %Power On
      (junction 913) -> Even_up_to_Odd.Main.Phase_B_Power_Off : %Power off
      Even_up_to_Odd.Main.Phase_B_Power_on -> Even_up_to_Odd.Main.Phase_C_Power_on : [CluOffTqTar<=0&&CluOnTqTar>=CluTqTarMax]
      Even_up_to_Odd.Main.Phase_B_Power_Off -> Even_up_to_Odd.Main.Phase_C_Power_Off : [CluOffTqTar<=0&&EngN<=CluOnN]
      Even_up_to_Odd.Main.Phase_C_Power_on -> Even_up_to_Odd.Main.Phase_D_Power_on : [abs(EngN-CluOnN)<50||...
          | EngN<=CluOnN]
      Even_up_to_Odd.Main.Phase_C_Power_Off -> Even_up_to_Odd.Main.Phase_D_Power_Off : [abs(EngN-CluOnN)<50||...
          | EngN>=CluOnN]
      Even_up_to_Odd.Main.Phase_D_Power_on -> Even_up_to_Odd.Main.Phase_E_Power_on : [abs(EngN-CluOnN)<10]
      Even_up_to_Odd.Main.Phase_D_Power_Off -> Even_up_to_Odd.Main.Phase_E_Power_Off : [abs(EngN-CluOnN)<10]
      Even_up_to_Odd.Main.Phase_E_Power_Off -> Even_up_to_Odd.Main.End1 : [CluOnTqTar>=CluTqTarMax]
      Even_up_to_Odd.Main.Phase_E_Power_on -> Even_up_to_Odd.Main.End : [CluOnTqTar>=CluTqTarMax]
      Even_up_to_Odd.Main.End -> (junction 914)
      Even_up_to_Odd.Main.End1 -> (junction 886)
      (junction 886) -> (junction 914)
    state Output [parallel]
      en,du:
      Clu1TqTar=CluOnTqTar;
      Clu2TqTar=CluOffTqTar;
      settings: executionOrder=3
    (junction 914) -> (junction 585)
  state Even_down_to_Odd
    state Input [parallel]
      % states initialized
      en:
      Clu1Act=0;
      Clu2Act=1;
      Clu1PReqFlg=1;
      Clu2PReqFlg=1;
      Clu1TqTar=0;
      Clu2TqTar=Clu2TqCpEstimd;
      CluTqTarMin=0;
      CluTqTarMax=40000;
      % torque target initialized
      en:
      CluOffTqTar=Clu2TqTar;
      CluOnTqTar=Clu1TqTar;
      % speed allocation
      en,du:
      CluOffN=InpShaft2N;
      CluOnN=InpShaft1N;
      settings: executionOrder=1
      note: Shift from even gear to odd gear,
          | clutch 1 as off-coming clutch,
          | clutch 2 as on-going clutch
    state Main [parallel]
      settings: executionOrder=2
      state Phase_A
        %Preparation
        state Phase_A_Off_Going [parallel]
          settings: executionOrder=1
          state Phase_A_Off_Going1
            %release to slip
            en,du:
            CluTqTarMin=0;
            CluTqDec=1000;
            CluOffTqTar=max(CluOffTqTar-CluTqDec,CluTqTarMin);
          state Phase_A_Off_Going2
            en,du:
            CluTqTarMin=0;
            CluTqDec=100;
            CluOffTqTar=max(CluOffTqTar-CluTqDec,CluTqTarMin);
          state Phase_A_Off_Going3
          (default) -> Even_down_to_Odd.Main.Phase_A.Phase_A_Off_Going.Phase_A_Off_Going1
          Even_down_to_Odd.Main.Phase_A.Phase_A_Off_Going.Phase_A_Off_Going1 -> Even_down_to_Odd.Main.Phase_A.Phase_A_Off_Going.Phase_A_Off_Going2 : [CluOffTqTar<EngTq]
          Even_down_to_Odd.Main.Phase_A.Phase_A_Off_Going.Phase_A_Off_Going2 -> Even_down_to_Odd.Main.Phase_A.Phase_A_Off_Going.Phase_A_Off_Going3 : [abs(EngN-CluOffN)>10]
        state Phase_A_On_Coming [parallel]
          settings: executionOrder=2
          state Phase_A_On_Coming1
            %Wait_for_KissPoint
            en:
            CluOnTqTar=1;
          (default) -> Even_down_to_Odd.Main.Phase_A.Phase_A_On_Coming.Phase_A_On_Coming1
      state Phase_B_Power_on
        %Inertia Phase, Handover
        state Phase_B_Off_Going [parallel]
          settings: executionOrder=2
          state Phase_B_Off_Going1
            en,du:
            CluTqTarMin=0;
            CluTqDec=500;
            CluOffTqTar=max(CluOffTqTar-CluTqDec,CluTqTarMin);
          (default) -> Even_down_to_Odd.Main.Phase_B_Power_on.Phase_B_Off_Going.Phase_B_Off_Going1
        state Phase_B_On_Coming [parallel]
          settings: executionOrder=1
      state Phase_B_Power_Off
        %Torque Phase, Handover
        state Phase_B_Off_Going [parallel]
          settings: executionOrder=2
          state Phase_B_Off_Going1
            en,du:
            CluTqTarMin=0;
            CluTqDec=550;
            CluOffTqTar=max(CluOffTqTar-CluTqDec,CluTqTarMin);
          (default) -> Even_down_to_Odd.Main.Phase_B_Power_Off.Phase_B_Off_Going.Phase_B_Off_Going1
        state Phase_B_On_Coming [parallel]
          settings: executionOrder=1
          state Phase_B_On_Coming1
            en,du:
            CluTqTarMax=Close_Torque_Target(EngThr);
            CluTqInc=500;
            CluOnTqTar=min(Clu2TqTar+CluTqInc,CluTqTarMax);
          (default) -> Even_down_to_Odd.Main.Phase_B_Power_Off.Phase_B_On_Coming.Phase_B_On_Coming1
      state Phase_C_Power_on
        %Torque Phase
        state Phase_C_Off_Going [parallel]
          settings: executionOrder=1
          state Phase_C_Off_Going1
          state Phase_C_Off_Going2
            en,du:
            CluTqTarMin=0;
            CluTqDec=550;
            CluOffTqTar=max(CluOffTqTar-CluTqDec,CluTqTarMin);
          (default) -> Even_down_to_Odd.Main.Phase_C_Power_on.Phase_C_Off_Going.Phase_C_Off_Going1
          Even_down_to_Odd.Main.Phase_C_Power_on.Phase_C_Off_Going.Phase_C_Off_Going1 -> Even_down_to_Odd.Main.Phase_C_Power_on.Phase_C_Off_Going.Phase_C_Off_Going2 : [CluOffTqTar+CluOnTqTar>=EngTq]
        state Phase_C_On_Coming [parallel]
          settings: executionOrder=2
          state Phase_C_On_Coming1
            en,du:
            CluTqTarMax=Close_Torque_Target(EngThr);
            CluTqInc=500;
            CluOnTqTar=min(CluOnTqTar+CluTqInc,CluTqTarMax);
          (default) -> Even_down_to_Odd.Main.Phase_C_Power_on.Phase_C_On_Coming.Phase_C_On_Coming1
      state Phase_C_Power_Off
        %Inertia Phase
        en,du:
        CluTqTarMax=Close_Torque_Target(EngThr);
        CluTqInc=500;
        CluOnTqTar=min(CluOnTqTar+CluTqInc,CluTqTarMax);
      state Phase_D_Power_on
        %Synchronization Moment
        en,du:
        CluTqTarMax=Close_Torque_Target(EngThr);
        CluTqInc=500;
        CluOnTqTar=min(CluOnTqTar+CluTqInc,CluTqTarMax);
      state Phase_D_Power_Off
        %Synchronization Moment
        en,du:
        CluTqTarMax=Close_Torque_Target(EngThr);
        CluTqInc=500;
        CluOnTqTar=min(CluOnTqTar+CluTqInc,CluTqTarMax);
      state Phase_E_Power_on
        %Increae pressure for safety
        en,du:
        CluTqTarMax=Close_Torque_Target(EngThr);
        CluTqInc=1000;
        CluOnTqTar=min(CluOnTqTar+CluTqInc,CluTqTarMax);
      state Phase_E_Power_Off
        %Increae pressure for safety
        en,du:
        CluTqTarMax=Close_Torque_Target(EngThr);
        CluTqInc=1000;
        CluOnTqTar=min(CluOnTqTar+CluTqInc,CluTqTarMax);
      state End
      state End1
      (default) -> Even_down_to_Odd.Main.Phase_A
      Even_down_to_Odd.Main.Phase_A -> (junction 1152) : [CluOffTqTar<=0||...
          | abs(EngN-CluOffN)>10]
      (junction 1152) -> (junction 1147) [order 2]
      (junction 1152) -> Even_down_to_Odd.Main.Phase_B_Power_on [order 1] : [EngN>CluOffN]
          | %Power On
      (junction 1147) -> Even_down_to_Odd.Main.Phase_B_Power_Off : %Power off
      Even_down_to_Odd.Main.Phase_B_Power_on -> Even_down_to_Odd.Main.Phase_B_Power_Off [order 2] : [EngTq<=0]
          | %change mind
          | % from power-on to power-off
      Even_down_to_Odd.Main.Phase_B_Power_on -> Even_down_to_Odd.Main.Phase_C_Power_on [order 1] : [EngN>CluOnN]
      Even_down_to_Odd.Main.Phase_B_Power_Off -> Even_down_to_Odd.Main.Phase_C_Power_Off : [CluOffTqTar<=0]
      Even_down_to_Odd.Main.Phase_C_Power_Off -> Even_down_to_Odd.Main.Phase_D_Power_Off : [abs(EngN-CluOnN)<50]
      Even_down_to_Odd.Main.Phase_C_Power_on -> Even_down_to_Odd.Main.Phase_D_Power_on : [CluOffTqTar<=0&&...
          | abs(EngN-CluOnN)<50]
      Even_down_to_Odd.Main.Phase_D_Power_on -> Even_down_to_Odd.Main.Phase_E_Power_on : [abs(EngN-CluOnN)<10]
      Even_down_to_Odd.Main.Phase_D_Power_Off -> Even_down_to_Odd.Main.Phase_E_Power_Off : [abs(EngN-CluOnN)<10]
      Even_down_to_Odd.Main.Phase_E_Power_Off -> Even_down_to_Odd.Main.End1 : [CluOnTqTar>=CluTqTarMax]
      Even_down_to_Odd.Main.Phase_E_Power_on -> Even_down_to_Odd.Main.End : [CluOnTqTar>=CluTqTarMax]
      Even_down_to_Odd.Main.End -> (junction 1142)
      Even_down_to_Odd.Main.End1 -> (junction 1132)
      (junction 1132) -> (junction 1142)
    state Output [parallel]
      en,du:
      Clu1TqTar=CluOnTqTar;
      Clu2TqTar=CluOffTqTar;
      settings: executionOrder=3
    (junction 1142) -> (junction 1188)
  Both_Off_from_Even2Odd.End -> Both_Clutch_Off
  (junction 97) -> Odd_up_to_Even [order 1] : [PreGearAct>GearAct]
  Odd_up_to_Even -> Both_Off_from_Odd2Even : [Clu1Req==0&&Clu2Req==0]
  (junction 97) -> Odd_down_to_Even [order 2] : [PreGearAct<GearAct]
  Drive_by_Odd -> (junction 97) [order 2] : [Clu1Req==0&&Clu2Req==1]
  Odd_down_to_Even -> Both_Off_from_Odd2Even : [Clu1Req==0&&Clu2Req==0]
  Even_Off.End -> Both_Clutch_Off
  (default) -> Both_Clutch_Off
  Even_On_Process.Even_On.End -> Drive_by_Even
  Drive_by_Odd -> Odd_Off [order 1] : [Clu1Req==0&&Clu2Req==0]
  Drive_by_Even -> Even_Off [order 1] : [Clu1Req==0&&Clu2Req==0]
  Odd_On_Process -> Odd_Off : [Clu1Req==0]
  Even_On_Process -> Even_Off : [Clu2Req==0]
  Both_Clutch_Off -> (junction 68) [order 1] : [(Clu1Req==1&&Clu2Req==0)&&...
      | EngN>EngNIdleMin]
  Both_Clutch_Off -> (junction 71) [order 2] : [(Clu1Req==0&&Clu2Req==1)&&...
      | EngN>EngNIdleMin]
  (junction 273) -> Drive_by_Odd
  (junction 428) -> Drive_by_Even
  (junction 71) -> Even_On [order 2]
  (junction 68) -> Odd_On [order 3]
  (junction 137) -> Drive_by_Odd
  (junction 68) -> Odd_Launch [order 2] : [GearAct==0&&...
      | PreGearAct==1]
  (junction 71) -> Even_Launch [order 1] : [GearAct==0&&...
      | PreGearAct==2]
  (junction 68) -> Reverse_Launch [order 1] : [GearAct==0&&...
      | PreGearAct==7]
  (junction 1009) -> Drive_by_Even
  Drive_by_Even -> (junction 107) [order 2] : [Clu1Req==1&&Clu2Req==0]
  Odd_Off.End -> Both_Clutch_Off
  (junction 585) -> Drive_by_Odd
  Even_down_to_Odd -> Both_Off_from_Even2Odd : [Clu1Req==0&&Clu2Req==0]
  Even_up_to_Odd -> Both_Off_from_Even2Odd : [Clu1Req==0&&Clu2Req==0]
  (junction 107) -> Even_up_to_Odd [order 1] : [PreGearAct>GearAct]
  (junction 107) -> Even_down_to_Odd [order 2] : [PreGearAct<GearAct]
  Odd_On_Process.Odd_On.End -> Drive_by_Odd
  (junction 859) -> Drive_by_Even
  (junction 1188) -> Drive_by_Odd
  Both_Off_from_Odd2Even.End -> Both_Clutch_Off
  data: AccPeld function_input double size=1; Inten function_output double size=1; TqOld function_input uint16 size=1; Inten function_input int16 size=1; EngN function_input int16 size=1; CluN function_input int16 size=1; TqNew function_output uint16; EngThr function_input uint8 size=1; Tq function_output uint16 size=1; EngThr function_input uint8 size=1; Tq function_output uint16 size=1; GearAct input uint8; PreGearAct input uint8; Clu1Req input uint8; Clu2Req input uint8; EngThr input uint8; EngTq input uint16; EngN input int16; InpShaft1N input int16; InpShaft2N input int16; Clu1TqCpEstimd input uint16; Clu2TqCpEstimd input uint16; AccPedl input uint8; Clu1Act output uint8; Clu2Act output uint8; Clu1TqTar output uint16; Clu2TqTar output uint16; Clu1PReqFlg output uint8; Clu2PReqFlg output uint8; EngTqIntvFlg output uint8; EngTqIntvRat output uint8; EngNIdle parameter uint16; VehSpd input uint16; CluNDifRng local int16; CluClsTqRatFast local uint16; CluTqTarMax local uint16; CluTqInc local uint16; CluTqDec local uint16; EngNIdleMin parameter uint16; CluTqTarMin local uint16; DrvrInten input int16; CluOffN local int16; CluOnN local int16; CluOffTqTar local uint16; CluOnTqTar local uint16
